simulink model "BAES_RAGUSANTE_Block_Diagram_Algebra_NUMBER1_REDUCED_Simulink"  (R2023b)
settings: Solver=VariableStepAuto  StartTime=0.0  StopTime=20.0  RelTol=1e-3
values from neighbouring files (symbols this model uses):
  TF_Final_den = conv (TF4_den, TF3TBR_den)    [BAES_RAGUSANTE_Block_Diagram_Algebra_NUMBER1_REDUCED.m]
  TF_Final_num = conv (TF4_num, TF3TBR_num)    [BAES_RAGUSANTE_Block_Diagram_Algebra_NUMBER1_REDUCED.m]
settings Model: Creator=EUNICE CHLOE  LastModifiedBy=EUNICE CHLOE

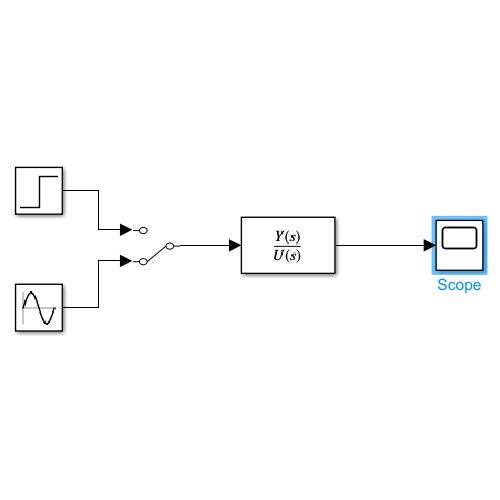
[thumbnail: Simulink's stored preview of the top-level diagram]
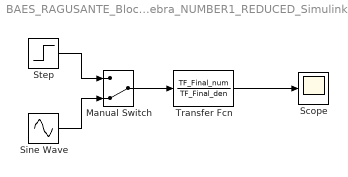
== system BAES_RAGUSANTE_Block_Diagram_Algebra_NUMBER1_REDUCED_Simulink ==
  Manual Switch : ManualSwitch  CurrentSetting=0
  Scope : Scope
  Sine Wave : Sin  SampleTime=0
  Step : Step  Time=0  SampleTime=0
  Transfer Fcn : TransferFcn  Numerator=TF_Final_num  Denominator=TF_Final_den
  wires:
  Step/1 -> Manual Switch/1
  Sine Wave/1 -> Manual Switch/2
  Manual Switch/1 -> Transfer Fcn/1
  Transfer Fcn/1 -> Scope/1
